simulink model "2R teleoperation system"  (R2017b)
settings: Solver=VariableStepAuto  StartTime=0.0  StopTime=10  MinStep=1e-40  RelTol=1e-4
settings Model: Creator=ANANDA RANGAN N  LastModifiedBy=ANANDA RANGAN N
settings SolverCC: ZeroCrossAlgorithm=Adaptive  AlgebraicLoopSolver=LineSearch

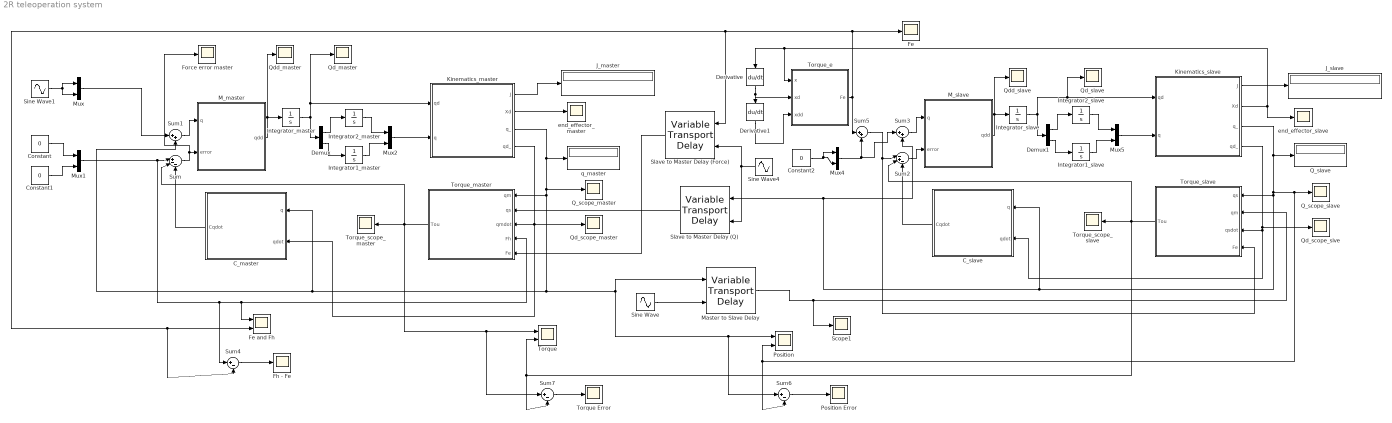
== system 2R teleoperation system ==
  C_master : MATLAB Function  TreatAsAtomicUnit=on
  C_slave : MATLAB Function  TreatAsAtomicUnit=on
  Constant : Constant  Value=0
  Constant1 : Constant  Value=0
  Constant2 : Constant  Value=0
  Demux : Demux  Outputs=2
  Demux1 : Demux  Outputs=2
  Derivative : Derivative
  Derivative1 : Derivative
  Fe : Scope
  Fe and Fh : Scope  NumInputPorts=2
  Fh - Fe : Scope
  Force error master : Scope
  Integrator1_master : Integrator
  Integrator1_slave : Integrator  InitialCondition=0.5
  Integrator2_master : Integrator
  Integrator2_slave : Integrator  InitialCondition=1
  Integrator_master : Integrator  IgnoreLimit=on
  Integrator_slave : Integrator
  J_master : Display
  J_slave : Display
  Kinematics_master : MATLAB Function  TreatAsAtomicUnit=on
  Kinematics_slave : MATLAB Function  TreatAsAtomicUnit=on
  M_master : MATLAB Function  TreatAsAtomicUnit=on
  M_slave : MATLAB Function  TreatAsAtomicUnit=on
  Master to Slave Delay : VariableTransportDelay  MaximumDelay=10  MaximumPoints=2048
  Mux{,1..2,4..5} (5 alike) : Mux  Inputs=2
  Position : Scope  NumInputPorts=2
  Position Error : Scope
  Q_scope_master : Scope
  Q_scope_slave : Scope
  Q_slave : Display
  Qd_master : Scope
  Qd_scope_master : Scope
  Qd_scope_slve : Scope
  Qd_slave : Scope
  Qdd_master : Scope
  Qdd_slave : Scope
  Scope1 : Scope
  Sine Wave : Sin  Amplitude=0.25  Bias=0.25  Frequency=0.1  SampleTime=0
  Sine Wave1 : Sin  Amplitude=0  Bias=1  SampleTime=0
  Sine Wave4 : Sin  Amplitude=0.25  Bias=0.25  Frequency=0.5  SampleTime=0
  Slave to Master Delay (Force) : VariableTransportDelay  MaximumDelay=10  MaximumPoints=2048
  Slave to Master Delay (Q) : VariableTransportDelay  MaximumDelay=10  MaximumPoints=2048
  Sum : Sum  Inputs=|+--
  Sum1 : Sum  Inputs=|++
  Sum2 : Sum  Inputs=|-+-
  Sum3 : Sum  Inputs=|++
  Sum4 : Sum  Inputs=|+-
  Sum5 : Sum  Inputs=|++
  Sum6 : Sum  Inputs=|+-
  Sum7 : Sum  Inputs=|+-
  Torque : Scope  NumInputPorts=2
  Torque Error : Scope
  Torque_e : MATLAB Function  TreatAsAtomicUnit=on
  Torque_master : MATLAB Function  TreatAsAtomicUnit=on
  Torque_scope_master : Scope
  Torque_scope_slave : Scope
  Torque_slave : MATLAB Function  TreatAsAtomicUnit=on
  end_effector_master : Scope
  end_effector_slave : Scope
  q_master : Display
  wires:
  Mux1/1 -> Sum4/1, Fe and Fh/1, Torque_master/4(Fh), Sum/1
  Sum/1 -> Force error master/1, M_master/2(error)
  C_master/1(Cqdot) -> Sum/3
  Demux/1 -> Integrator2_master/1
  Demux/2 -> Integrator1_master/1
  Integrator1_master/1 -> Mux2/2
  Integrator2_master/1 -> Mux2/1
  Mux2/1 -> Kinematics_master/2(q)
  Sum1/1 -> M_master/1(q)
  Kinematics_master/3(q_) -> Torque_master/1(qm), Sum1/2, C_master/1(q), Sum6/1, Position/1, Master to Slave Delay/1, Q_scope_master/1, q_master/1
  Torque_master/1(Tou) -> Sum7/1, Torque/1, Torque_scope_master/1, Sum/2
  Kinematics_master/1(J) -> J_master/1
  Kinematics_master/2(Xd) -> end_effector_master/1
  C_slave/1(Cqdot) -> Sum2/3
  Sum2/1 -> M_slave/2(error)
  Sum5/1 -> Torque_slave/4(Fe), Sum2/1
  M_slave/1(qdd) -> Integrator_slave/1, Qdd_slave/1
  Kinematics_slave/1(J) -> J_slave/1
  Sum3/1 -> M_slave/1(q)
  Integrator_slave/1 -> Demux1/1, Qd_slave/1, Kinematics_slave/1(qd)
  Integrator2_slave/1 -> Mux5/1
  Demux1/2 -> Integrator1_slave/1
  Torque_slave/1(Tou) -> Sum7/2, Torque/2, Torque_scope_slave/1, Sum2/2
  Kinematics_slave/4(qd_) -> Torque_slave/3(qsdot), C_slave/2(qdot), Qd_scope_slve/1
  Mux5/1 -> Kinematics_slave/2(q)
  Demux1/1 -> Integrator2_slave/1
  Integrator1_slave/1 -> Mux5/2
  Kinematics_slave/3(q_) -> Q_scope_slave/1, Sum6/2, Position/2, Torque_slave/1(qs), Slave to Master Delay (Q)/1, Sum3/2, C_slave/1(q), Q_slave/1
  Sine Wave/1 -> Master to Slave Delay/2
  Sine Wave1/1 -> Mux/1, Mux/2
  Sine Wave4/1 -> Slave to Master Delay (Q)/2, Slave to Master Delay (Force)/2
  Slave to Master Delay (Force)/1 -> Torque_master/5(Fe)
  Slave to Master Delay (Q)/1 -> Torque_master/2(qs)
  Master to Slave Delay/1 -> Scope1/1, Torque_slave/2(qm)
  Integrator_master/1 -> Demux/1, Qd_master/1, Kinematics_master/1(qd)
  Kinematics_slave/2(Xd) -> end_effector_slave/1, Torque_e/1(x), Derivative/1
  Derivative1/1 -> Torque_e/3(xdd)
  Constant/1 -> Mux1/1
  Constant1/1 -> Mux1/2
  Derivative/1 -> Torque_e/2(xd), Derivative1/1
  Constant2/1 -> Mux4/2, Mux4/1
  Torque_e/1(Fe) -> Fe/1, Sum4/2, Fe and Fh/2, Slave to Master Delay (Force)/1, Sum5/1
  Mux4/1 -> Sum3/1, Sum5/2
  Sum6/1 -> Position Error/1
  Sum7/1 -> Torque Error/1
  M_master/1(qdd) -> Qdd_master/1, Integrator_master/1
  Kinematics_master/4(qd_) -> C_master/2(qdot), Qd_scope_master/1, Torque_master/3(qmdot)
  Mux/1 -> Sum1/1
  Sum4/1 -> Fh - Fe/1

== matlab function 2R teleoperation system/Kinematics_master ==
  data: qd input; q input; J output; Xd output; q_ output; qd_ output
function [J, Xd, q_, qd_] = fcn(qd, q)
 q1 = q(1);
 q2 = q(2);
 
 l = 0.18;
 
 if q1 < 0
    q1 = 0;
end

if q2 < 0
    q2 = 0;
end

if q1 >= pi
    q1 = pi;
end

if q2 >= pi
    q2 = pi;
end

x = l*(cos(q1) + cos(q1+q2));
y = l*(sin(q1) + sin(q1+q2));

dx1 = -l*(sin(q1)+sin(q1+q2));
dx2 = -l*sin(q1+q2);
dy1 = l*(cos(q1) + cos(q1+q2));
dy2 = l*cos(q1+q2);

Xd = [x; y];

J = [dx1 dx2; dy1 dy2];

%{
if qd(1) <= -100
    qd(1) = -100;
end

if qd(2) <= -100
    qd(2) = -100;
end

if qd(2) > 100
    qd(2) = 100;
end
    
if qd(1) > 100
    qd(1) = 100;
end
%}
qd_ = qd;
q(1) = q1;
q(2) = q2;
q_ = q;

== matlab function 2R teleoperation system/M_master ==
  data: q input; qdd output; error input
function qdd  = fcn(q, error)
 q1 = q(1);
 q2 = q(2); 
 
 m1 = 0.03;
 m2 = 0.03;
 
 l = 0.18;
 lc = 0.09;
 
 Jv1 = [-(lc)*sin(q1) 0; (lc)*cos(q1) 0];
 Jv2 = [-(l)*sin(q1)-(lc)*sin(q1+q2) -(lc)*sin(q1+q2); (l)*cos(q1)+(lc)*cos(q1+q2) (lc)*cos(q1+q2)];
 
 %M = m1*(Jv1')*(Jv1) + m2*(Jv2')*(Jv2);
 M= [(m1+m2)*(l^2)+(m2)*(l^2)+2*m2*(l^2)*cos(q2) m2*(l^2)+m2*(l^2)*cos(q2); 
       m2*(l^2)+m2*(l^2)*cos(q2) m2*(l^2)];
 
 g = 9.81;
 G = [(m2*l*g*cos(q1+q2))+(l*(m1+m2)*cos(q1)); g*l*m2*cos(q1+q2)];
 Minv = inv(M);
 
 %qdd = Minv*(error-G);

 qdd = Minv*(error);

== matlab function 2R teleoperation system/Torque_master ==
  data: qm input; qs input; qmdot input; Fh input; Tou output; Fe input
function Tou = fcn(qm, qs, qmdot, Fh, Fe)
Km = 0.9*[1 0; 0 1];
Pm = [1 0; 0 1];
E = 0.000019899999*[1;1];

Tou = Km*qmdot + Pm*(qm-qs) + Fh + (sign(qmdot)+E)*((Fh-Fe)')*(Fh-Fe) ;

== matlab function 2R teleoperation system/C_master ==
  data: q input; Cqdot output; qdot input
function Cqdot = fcn(q, qdot)
q1 = q(1);
q2 = q(2);

qd1 = qdot(1);
qd2 = qdot(2);

m1 = 0.03;
m2 = 0.03;
 
l = 0.18;
lc = 0.09;

C = [-2*l*l*m2*sin(q2)*qdot(2), -l*l*m2*sin(q2)*qdot(2); l*l*m2*sin(q2)*qdot(1), 0];
Cqdot = C*qdot;
%Cqdot = [-m2*(l^2)*sin(q2)*(2*qd2*qd1+(qd2^2)); -m2*(l^2)*sin(q2)*(q1^2)];
%error = [0 0; 0 0];
%Cqdot = [0;0];
%Cqdot = error * Cqdot;

== matlab function 2R teleoperation system/C_slave ==
  data: q input; Cqdot output; qdot input
function Cqdot = fcn(q, qdot)
q1 = q(1);
q2 = q(2);

qd1 = qdot(1);
qd2 = qdot(2);

m1 = 0.03;
m2 = 0.03;
 
l = 0.18;
lc = 0.09;
 
C=[-2*m2*(l^2)*sin(q2)*qd1, -m2*(l^2)*sin(q2)*qd2; m2*(l^2)*sin(q2)*qd1, 0];
Cqdot = C*qdot;
%Cqdot = [-m2*(l^2)*sin(q2)*(2*qd2*qd1 + (qd2^2)); -m2*(l^2)*sin(q2)*(q1^2)];

== matlab function 2R teleoperation system/Kinematics_slave ==
  data: qd input; q input; J output; Xd output; q_ output; qd_ output
function [J, Xd, q_, qd_] = fcn(qd, q)
 q1 = q(1);
 q2 = q(2);
 
 l = 0.18;
 
 if q1 < 0
    q1 = 0;
end

if q2 < 0
    q2 = 0;
end

if q1 >= pi
    q1 = pi;
end

if q2 >= pi
    q2 = pi;
end

x = l*(cos(q1) + cos(q1+q2));
y = l*(sin(q1) + sin(q1+q2));

dx1 = -l*(sin(q1)+sin(q1+q2));
dx2 = -l*sin(q1+q2);
dy1 = l*(cos(q1) + cos(q1+q2));
dy2 = l*cos(q1+q2);

Xd = [x; y];

J = [dx1 dx2; dy1 dy2];

%{
if qd(1) <= -100
    qd(1) = -100;
end

if qd(2) <= -100
    qd(2) = -100;
end

if qd(2) > 100
    qd(2) = 100;
end
    
if qd(1) > 100
    qd(1) = 100;
end
%}
qd_ = qd;
q(1) = q1;
q(2) = q2;
q_ = q;

== matlab function 2R teleoperation system/M_slave ==
  data: q input; qdd output; error input
function qdd  = fcn(q, error)
 q1 = q(1);
 q2 = q(2); 
 
 m1 = 0.03;
 m2 = 0.03;
 
 l = 0.18;
 lc = 0.09;


 Jv1 = [-(lc)*sin(q1) 0; (lc)*cos(q1) 0];
 Jv2 = [-(l)*sin(q1)-(lc)*sin(q1+q2) -(lc)*sin(q1+q2); (l)*cos(q1)+(lc)*cos(q1+q2) (lc)*cos(q1+q2)];
 
 %M = (Jv1')*m1*(Jv1) + (Jv2')*m2*(Jv2);
 M = [(m1+m2)*(l^2)+(m2)*(l^2)+2*m2*(l^2)*cos(q2) m2*(l^2)+m2*(l^2)*cos(q2); 
       m2*(l^2)+m2*(l^2)*cos(q2) m2*(l^2)];
 g = 9.81;
 G = [m2*l*g*cos(q1+q2)+ l*(m1+m2)*cos(q1); g*l*m2*cos(q1+q2)];
  
 Minv = inv(M);
 
 %qdd = Minv*(error-G);

 qdd = Minv*(error);

== matlab function 2R teleoperation system/Torque_slave ==
  data: qs input; qm input; qsdot input; Fe input; Tou output
function Tou = fcn(qs, qm, qsdot, Fe)
Ks = 0.9*[1 0; 0 1];
Ps = [1 0; 0 1];
Tou = -Ks*qsdot - Ps*(qs-qm) + Fe;

== matlab function 2R teleoperation system/Torque_e ==
  data: x input; xd input; xdd input; Fe output
function Fe = fcn(x, xd, xdd)
 Me = 0.5*[1 0; 0 1];
 Be = 0.15*[1 0; 0 1];
 Ke = 0.1*[1 0; 0 1];
 Fe = Be*xd + Ke*x;% + Me*xdd;
 
% Fe = [0; 0];
